simulink model "Inverters_control_error_ETR07"  (R2017b)
settings: Solver=FixedStepAuto  StartTime=0.0  StopTime=10.0  RelTol=1e-3
settings Model: Creator=cspt  LastModifiedBy=cspt
settings RTWCC: SystemTargetFile=irt.tlc  TemplateMakefile=irt_default_tmf  Description=INTECRIO Real-Time Target
settings STFCustomTargetCC: TargetLangStandard=C99 (ISO)  UtilityFuncGeneration=Shared location  SystemTargetFile=irt.tlc
settings GRTTargetCC: UtilityFuncGeneration=Shared location  ParMdlRefBuildCompliant=off  CompOptLevelCompliant=off  ConcurrentExecutionCompliant=off  CombineOutputUpdateFcns=off  MatFileLogging=off  CPPClassGenCompliant=off  GRTInterface=on  UseToolchainInfoCompliant=off  GenerateASAP2=on

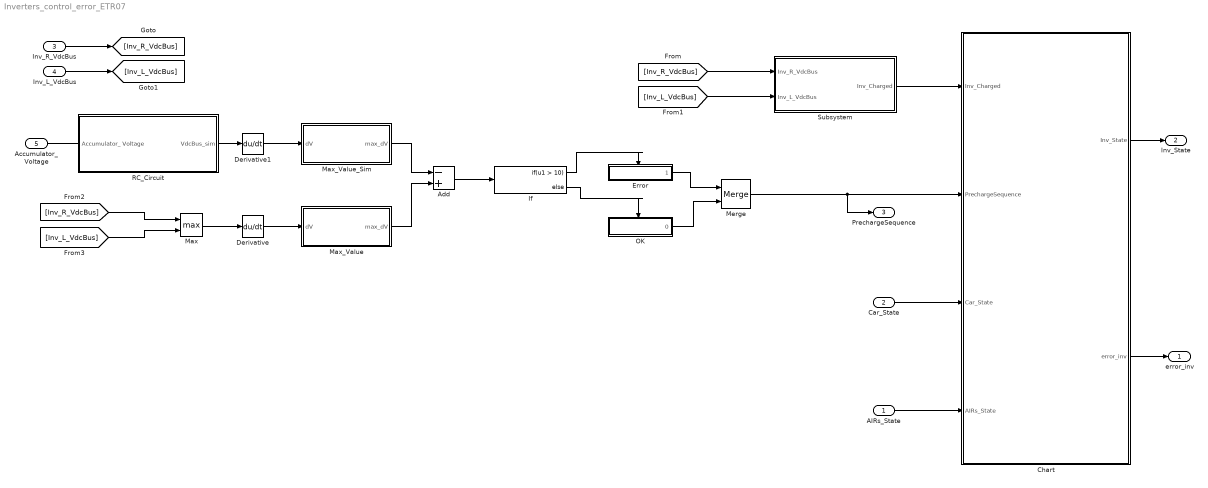
== system Inverters_control_error_ETR07 ==
  AIRs_State : Inport
  Car_State : Inport  Port=2
  Inv_R_VdcBus : Inport  Port=3
  Inv_L_VdcBus : Inport  Port=4
  Accumulator_Voltage : Inport  Port=5
  Add : Sum  Inputs=-+
  Chart : Stateflow chart  TreatAsAtomicUnit=on
  Derivative : Derivative
  Derivative1 : Derivative
  Error : Subsystem  TreatAsAtomicUnit=on
  If : If  IfExpression=u1 > 10
  Max : MinMax  Function=max  Inputs=2
  Max_Value : MATLAB Function  TreatAsAtomicUnit=on
  Max_Value_Sim : MATLAB Function  TreatAsAtomicUnit=on
  Merge : Merge
  OK : Subsystem  TreatAsAtomicUnit=on
  RC_Circuit : Subsystem
  Subsystem : Subsystem
  error_inv : Outport
  Inv_State : Outport  Port=2
  PrechargeSequence : Outport  Port=3
  wires:
  [Inv_L_VdcBus] -> Subsystem/2(Inv_L_VdcBus)
  [Inv_R_VdcBus] -> Subsystem/1(Inv_R_VdcBus)
  Subsystem/1(Inv_Charged) -> Chart/1(Inv_Charged)
  AIRs_State/1 -> Chart/4(AIRs_State)
  Chart/2(error_inv) -> error_inv/1
  Chart/1(Inv_State) -> Inv_State/1
  Inv_R_VdcBus/1 -> [Inv_R_VdcBus]
  Inv_L_VdcBus/1 -> [Inv_L_VdcBus]
  [Inv_L_VdcBus] -> Max/2
  [Inv_R_VdcBus] -> Max/1
  Max/1 -> Derivative/1
  Accumulator_Voltage/1 -> ?
  RC_Circuit/1(VdcBus_sim) -> Derivative1/1
  Derivative1/1 -> Max_Value_Sim/1(dV)
  Derivative/1 -> Max_Value/1(dV)
  Max_Value/1(max_dV) -> Add/2
  Max_Value_Sim/1(max_dV) -> Add/1
  Add/1 -> If/1
  If/1 -> Error/Action
  If/2 -> OK/Action
  OK/1(0) -> Merge/2
  Error/1(1) -> Merge/1
  Merge/1 -> PrechargeSequence/1, Chart/2(PrechargeSequence)
  Car_State/1 -> Chart/3(Car_State)

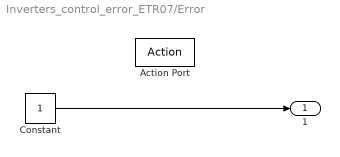
== system Inverters_control_error_ETR07/Error ==
  Action Port : ActionPort  ActionType=then
  Constant : Constant
  1 : Outport
  wires:
  Constant/1 -> 1/1

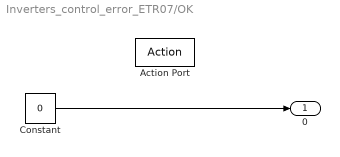
== system Inverters_control_error_ETR07/OK ==
  Action Port : ActionPort  ActionType=else
  Constant : Constant  Value=0
  0 : Outport
  wires:
  Constant/1 -> 0/1

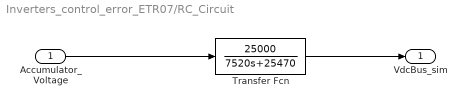
== system Inverters_control_error_ETR07/RC_Circuit ==
  Accumulator_ Voltage : Inport
  Transfer Fcn : TransferFcn  Numerator=[25000]  Denominator=[7520 25470]
  VdcBus_sim : Outport
  wires:
  Accumulator_ Voltage/1 -> Transfer Fcn/1
  Transfer Fcn/1 -> VdcBus_sim/1

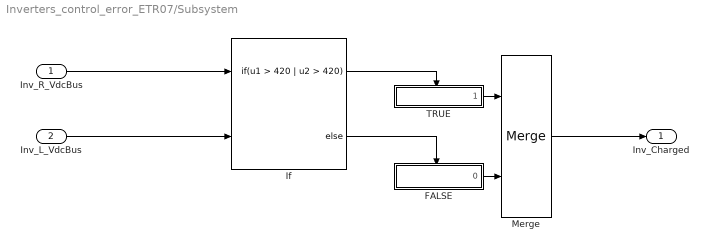
== system Inverters_control_error_ETR07/Subsystem ==
  Inv_R_VdcBus : Inport
  Inv_L_VdcBus : Inport  Port=2
  FALSE : Subsystem  TreatAsAtomicUnit=on
  If : If  NumInputs=2  IfExpression=u1 > 420 | u2 > 420
  Merge : Merge
  TRUE : Subsystem  TreatAsAtomicUnit=on
  Inv_Charged : Outport
  wires:
  Inv_L_VdcBus/1 -> If/2
  Inv_R_VdcBus/1 -> If/1
  If/2 -> FALSE/Action
  Merge/1 -> Inv_Charged/1
  If/1 -> TRUE/Action
  TRUE/1(1) -> Merge/1
  FALSE/1(0) -> Merge/2

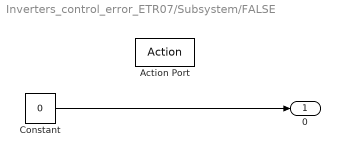
== system Inverters_control_error_ETR07/Subsystem/FALSE ==
  Action Port : ActionPort  ActionType=else
  Constant : Constant  Value=0
  0 : Outport
  wires:
  Constant/1 -> 0/1

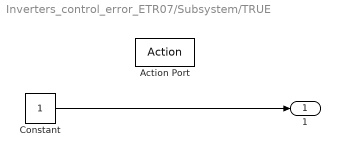
== system Inverters_control_error_ETR07/Subsystem/TRUE ==
  Action Port : ActionPort  ActionType=then
  Constant : Constant
  1 : Outport
  wires:
  Constant/1 -> 1/1

== matlab function Inverters_control_error_ETR07/Max_Value_Sim ==
  settings: updateMethod=DISCRETE
  data: dV input; max_dV output
function max_dV  = max_val(dV)

persistent dVpre

if isempty(dVpre)
    dVpre = 0;
end

if (dVpre > dV)
    max_dV = dVpre;
else
    max_dV = dV;
end
dVpre = max_dV;

== matlab function Inverters_control_error_ETR07/Max_Value ==
  settings: updateMethod=DISCRETE
  data: dV input; max_dV output
function max_dV  = max_val(dV)

persistent dVpre

if isempty(dVpre)
    dVpre = 0;
end

if (dVpre > dV)
    max_dV = dVpre;
else
    max_dV = dV;
end
dVpre = max_dV;

== stateflow chart Inverters_control_error_ETR07/Chart ==
  state InvDischarged
    entry: Inv_State = 0;
  state FAIL [group]
    state InvChargingError
      entry: Inv_State = 21;
    state OpenHVDBox
      entry: Inv_State = 24;
    InvChargingError -> OpenHVDBox : [AIRs_State == 0 & after(5, sec) & Inv_Charged == 1]{error_inv == 6}
  state InvCharging
    entry: Inv_State = 3;
  state InvCharged
    entry: Inv_State = 6;
  (default) -> InvDischarged : {error_inv=0}
  InvDischarged -> InvChargingError [order 2] : [AIRs_State == 6 & PrechargeSequence == 1]{error_inv==3}
  OpenHVDBox -> InvDischarged : [ Car_State == 0]
  InvDischarged -> InvCharging [order 1] : [AIRs_State == 6 & PrechargeSequence == 0]
  InvCharging -> InvChargingError [order 2] : [PrechargeSequence == 1 & Car_State == 9]
  InvCharging -> InvCharged [order 1] : [AIRs_State == 3 & Inv_Charged == 1 & PrechargeSequence == 0]
  InvCharged -> OpenHVDBox : [AIRs_State == 0 & after(5, sec) & Inv_Charged == 1]{error_inv == 6}
  data: Inv_Charged input; PrechargeSequence input; Car_State input; AIRs_State input; Inv_State output; error_inv output
